simulink model "SVFB_notclean"  (R2024a)
settings: Solver=ode45  StartTime=0.0  StopTime=3  RelTol=1e-3
undefined symbols (not defined in the file): A, B, C, closed_loop_dynamics, closed_loop_observer, K0, L_luemb, S0_x0, Si_x0
settings Model: Creator=aless  LastModifiedBy=Stefano

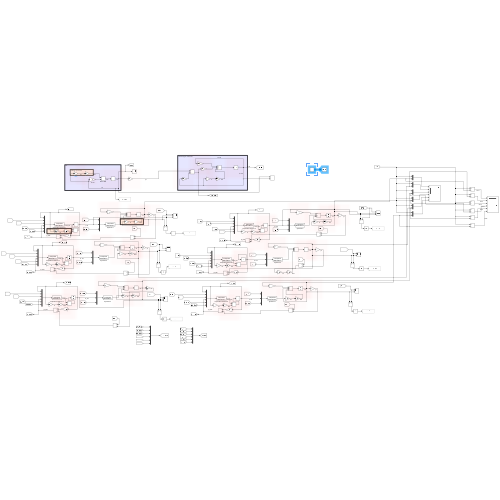
[thumbnail: Simulink's stored preview of the top-level diagram]
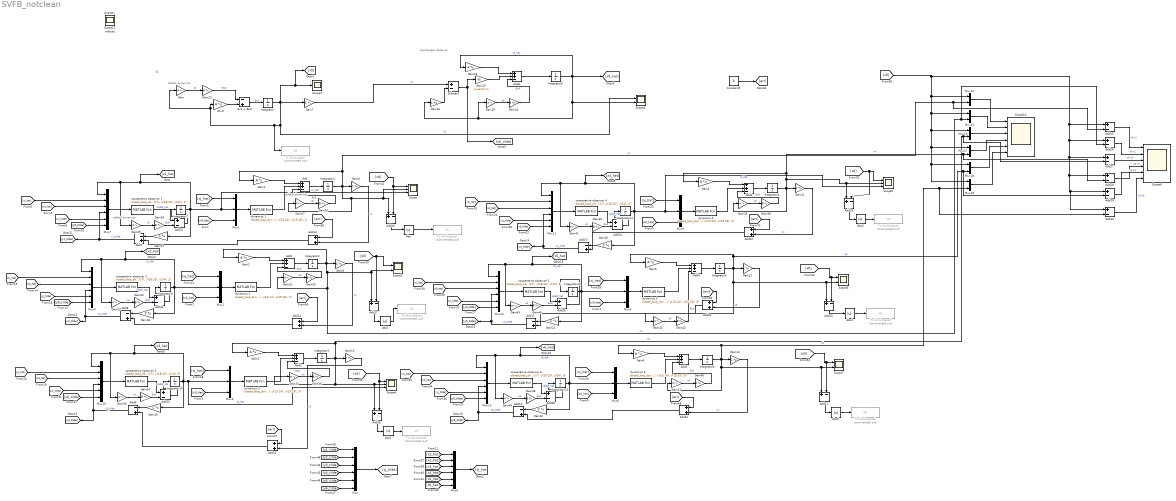
== system SVFB_notclean ==
  note: luemberger observer
  note: S0
  note: added dynamics
  note: added dynamics
  note: added dynamics
  A*x0 : Gain  Gain=A  Multiplication=Matrix(K*u)
  Abs{,1..5} (6 alike) : Abs  SaturateOnIntegerOverflow=off
  Add{,1..6} (7 alike) : Sum  Inputs=++-
  Add{7..12} (6 alike) : Sum  Inputs=-+
  Add{13..15,22..24} (6 alike) : Sum
  Add{16..21,25..36} (18 alike) : Sum  Inputs=+-
  Ax0 + Bu0 : Sum  Inputs=-+
  Constant5 : Constant  Value=0
  Gain{,25,27,29,31,33,35,37,39,41,43,45,47,49} (14 alike) : Gain  Gain=K0  Multiplication=Matrix(K*u)
  Gain{1..6,14} (7 alike) : Gain  Gain=A  Multiplication=Matrix(K*u)
  Gain{7..13,16..22} (14 alike) : Gain  Gain=C  Multiplication=Matrix(K*u)
  Gain15 : Gain  Gain=L_luemb  Multiplication=Matrix(K*u)
  Gain{23..24,26,28,30,32,34,36,38,40,42,44,46,48} (14 alike) : Gain  Gain=B  Multiplication=Matrix(K*u)
  Integrator : Integrator  InitialCondition=S0_x0
  Integrator{1..7,9..13} (12 alike) : Integrator  InitialCondition=Si_x0
  Integrator8 : Integrator  InitialCondition=S0_x0
  Mux{,7..13} (8 alike) : Mux  Inputs=6
  Mux{1..6} (6 alike) : Mux  Inputs=3
  Mux{14..19} (6 alike) : Mux  Inputs=2
  Scope : Scope  NumInputPorts=3
  Scope1 : Scope
  Scope10 : Scope  NumInputPorts=6
  Scope{2..3,6..7} (4 alike) : Scope  NumInputPorts=2
  Scope4 : Scope  NumInputPorts=3
  Scope5 : Scope  NumInputPorts=3
  Scope8 : Scope  NumInputPorts=6
  Subtract : Sum  Inputs=+-
  To Workspace1 : ToWorkspace  Commented=on  VariableName=x1  SaveFormat=Timeseries  SampleTime=-1
  To Workspace2 : ToWorkspace  Commented=on  VariableName=x2  SaveFormat=Timeseries  SampleTime=-1
  To Workspace3 : ToWorkspace  Commented=on  VariableName=x3  SaveFormat=Timeseries  SampleTime=-1
  To Workspace4 : ToWorkspace  Commented=on  VariableName=x4  SaveFormat=Timeseries  SampleTime=-1
  To Workspace5 : ToWorkspace  Commented=on  VariableName=x5  SaveFormat=Timeseries  SampleTime=-1
  To Workspace6 : ToWorkspace  Commented=on  VariableName=x6  SaveFormat=Timeseries  SampleTime=-1
  To Workspace7 : ToWorkspace  Commented=on  VariableName=x0  SampleTime=-1
  cooperative observer 1 : MATLABFcn  MATLABFcn=closed_loop_observer(u(1:2), u(3:14), u(15:16), u(17), u(18:23), u(24), 1)
  cooperative observer 2 : MATLABFcn  MATLABFcn=closed_loop_observer(u(1:2), u(3:14), u(15:16), u(17), u(18:23), u(24), 2)
  cooperative observer 3 : MATLABFcn  MATLABFcn=closed_loop_observer(u(1:2), u(3:14), u(15:16), u(17), u(18:23), u(24), 3)
  cooperative observer 4 : MATLABFcn  MATLABFcn=closed_loop_observer(u(1:2), u(3:14), u(15:16), u(17), u(18:23), u(24), 4)
  cooperative observer 5 : MATLABFcn  MATLABFcn=closed_loop_observer(u(1:2), u(3:14), u(15:16), u(17), u(18:23), u(24), 5)
  cooperative observer 6 : MATLABFcn  MATLABFcn=closed_loop_observer(u(1:2), u(3:14), u(15:16), u(17), u(18:23), u(24), 6)
  dynamics 1 : MATLABFcn  MATLABFcn=closed_loop_dynamics(u(1:12), u(13:14), u(15:16), 1)
  dynamics 2 : MATLABFcn  MATLABFcn=closed_loop_dynamics(u(1:12), u(13:14), u(15:16), 2)
  dynamics 3 : MATLABFcn  MATLABFcn=closed_loop_dynamics(u(1:12), u(13:14), u(15:16), 3)
  dynamics 4 : MATLABFcn  MATLABFcn=closed_loop_dynamics(u(1:12), u(13:14), u(15:16), 4)
  dynamics 5 : MATLABFcn  MATLABFcn=closed_loop_dynamics(u(1:12), u(13:14), u(15:16), 5)
  dynamics 6 : MATLABFcn  MATLABFcn=closed_loop_dynamics(u(1:12), u(13:14), u(15:16), 6)
  Scope11 : Scope
  position : Scope
  velocity : Scope
  wires:
  A*x0/1 -> Ax0 + Bu0/2
  Integrator8/1 -> Gain14/1, [x0_hat], Gain25/1, Gain16/1, Scope2/2  "x0_hat"
  Add6/1 -> Integrator8/1
  Gain7/1 -> Subtract/1  "y0"
  Gain15/1 -> Add6/2
  Subtract/1 -> [y0_tilde], Gain15/1
  Ax0 + Bu0/1 -> Integrator/1  "dx0"
  Integrator/1 -> [x0], Scope1/1, Gain7/1, Scope2/1, To Workspace7/1, Gain/1, A*x0/1  "x0"
  Gain14/1 -> Add6/1
  Gain16/1 -> Subtract/2
  Gain21/1 -> Add11/1
  Add12/1 -> [y6_tilde], Mux13/4  "y6_tilde"
  Add7/1 -> [y1_tilde], Mux7/4  "y1_tilde"
  [y5_tilde] -> Mux/5
  Gain19/1 -> Add9/1
  Gain22/1 -> Add12/1
  Mux10/1 -> cooperative observer 3/1
  [y0_tilde] -> Mux10/6
  Add2/1 -> Integrator3/1
  Integrator10/1 -> Gain19/1, [x3_hat], Gain35/1, Mux10/1, Scope4/3, Mux3/2  "x3_hat"
  [x0_hat] -> Mux3/3
  [x0_hat] -> Mux10/3
  Mux3/1 -> dynamics 3/1
  Integrator3/1 -> Add27/2, Mux16/2, Gain3/1, Gain37/1, Add18/1, Scope4/2, Gain10/1  "x3"
  dynamics 3/1 -> Add2/2
  [yj_tilde] -> Mux10/5
  Mux11/1 -> cooperative observer 4/1
  [xj_hat] -> Mux4/1
  Mux4/1 -> dynamics 4/1
  [y0_tilde] -> Mux11/6
  Gain3/1 -> Add2/1
  Integrator4/1 -> Gain11/1, Gain39/1, Add28/2, Mux17/2, Gain4/1, Add19/1, Scope5/2  "x4"
  Add3/1 -> Integrator4/1
  Integrator11/1 -> Gain20/1, [x4_hat], Gain41/1, Mux11/1, Scope5/3, Mux4/2  "x4_hat"
  dynamics 4/1 -> Add3/2
  Gain4/1 -> Add3/1
  [yj_tilde] -> Mux11/5
  Mux12/1 -> cooperative observer 5/1
  [xj_hat] -> Mux5/1
  Add4/1 -> Integrator5/1
  Integrator12/1 -> Gain21/1, [x5_hat], Gain45/1, Mux12/1, Mux5/2  "x5_hat"
  [x0_hat] -> Mux12/3
  dynamics 5/1 -> Add4/2
  Integrator5/1 -> Gain43/1, Scope6/2, Add20/1, Add29/2, Mux18/2, Gain5/1, Gain12/1  "x5"
  [xj_hat] -> Mux12/2
  [x0_hat] -> Mux5/3
  [yj_tilde] -> Mux12/5
  [x5_hat] -> Mux8/5
  [x3_hat] -> Mux8/3
  [x0_hat] -> Mux11/3
  [x2_hat] -> Mux8/2
  Gain18/1 -> Add8/1
  [yj_tilde] -> Mux9/5
  dynamics 2/1 -> Add1/2
  Gain2/1 -> Add1/1
  Integrator2/1 -> Gain31/1, Add26/2, Mux15/2, Scope3/2, Add17/1, Gain2/1, Gain9/1  "x2"
  Add10/1 -> Mux11/4, [y4_tilde]  "y4_tilde"
  Mux2/1 -> dynamics 2/1
  Gain5/1 -> Add4/1
  [x0_hat] -> Mux9/3
  [x0_hat] -> Mux2/3
  [xj_hat] -> Mux9/2
  Add11/1 -> Mux12/4, [y5_tilde]  "y5_tilde"
  [xj_hat] -> Mux2/1
  [y0_tilde] -> Mux9/6
  Integrator9/1 -> Gain18/1, [x2_hat], Gain33/1, Mux9/1, Mux2/2  "x2_hat"
  Add1/1 -> Integrator2/1
  Add5/1 -> Integrator6/1
  Mux13/1 -> cooperative observer 6/1
  [x0_hat] -> Mux4/3
  Integrator13/1 -> Gain22/1, [x6_hat], Gain49/1, Mux13/1, Mux6/2  "x6_hat"
  [x0_hat] -> Mux6/3
  [y0_tilde] -> Mux13/6
  Mux9/1 -> cooperative observer 2/1
  Mux6/1 -> dynamics 6/1
  [xj_hat] -> Mux6/1
  Integrator6/1 -> Gain47/1, Add21/1, Scope7/2, Add30/2, Mux19/2, Gain6/1, Gain13/1  "x6"
  Gain20/1 -> Add10/1
  [x6_hat] -> Mux8/6
  [y6_tilde] -> Mux/6
  Add8/1 -> [y2_tilde], Mux9/4  "y2_tilde"
  [yj_tilde] -> Mux13/5
  [y4_tilde] -> Mux/4
  Add9/1 -> [y3_tilde], Mux10/4  "y3_tilde"
  [y1_tilde] -> Mux/1
  Gain6/1 -> Add5/1
  Mux5/1 -> dynamics 5/1
  Mux7/1 -> cooperative observer 1/1
  [y3_tilde] -> Mux/3
  [y0_tilde] -> Mux12/6
  [xj_hat] -> Mux7/2
  [xj_hat] -> Mux3/1
  [x0_hat] -> Mux1/3
  [y0_tilde] -> Mux7/6
  Gain17/1 -> Add7/1
  [xj_hat] -> Mux1/1
  Mux8/1 -> [xj_hat]
  [x1_hat] -> Mux8/1
  [y2_tilde] -> Mux/2
  dynamics 6/1 -> Add5/2
  Integrator7/1 -> Gain17/1, [x1_hat], Gain29/1, Mux7/1, Scope/3, Mux1/2  "x1_hat"
  [xj_hat] -> Mux13/2
  [x0] -> Scope/1, Add16/2
  [xj_hat] -> Mux10/2
  [x0_hat] -> Mux7/3
  Integrator1/1 -> Gain27/1, Add16/1, Scope/2, Add25/2, Mux14/2, Gain1/1, Gain8/1  "x1"
  dynamics 1/1 -> Add/2
  [x4_hat] -> Mux8/4
  Add/1 -> Integrator1/1
  [x0_hat] -> Mux13/3
  Mux1/1 -> dynamics 1/1
  Gain1/1 -> Add/1
  [xj_hat] -> Mux11/2
  [yj_tilde] -> Mux7/5
  [x0] -> Scope3/1, Add17/2
  [x0] -> Add18/2, Scope4/1
  [x0] -> Add19/2, Scope5/1
  [x0] -> Scope6/1, Add20/2
  [x0] -> Add21/2, Scope7/1
  Mux/1 -> [yj_tilde]
  Mux14/1 -> Scope10/1
  Mux15/1 -> Scope10/2
  Mux16/1 -> Scope10/3
  Mux17/1 -> Scope10/4
  Mux18/1 -> Scope10/5
  Mux19/1 -> Scope10/6
  [x0] -> Add30/1, Add29/1, Add28/1, Add27/1, Add26/1, Add25/1, Mux19/1, Mux18/1, Mux17/1, Mux16/1, Mux15/1, Mux14/1
  Add16/1 -> Abs/1
  Abs/1 -> To Workspace1/1
  Add17/1 -> Abs1/1
  Abs1/1 -> To Workspace2/1
  Add18/1 -> Abs2/1
  Abs2/1 -> To Workspace3/1
  Add19/1 -> Abs3/1
  Abs3/1 -> To Workspace4/1
  Add20/1 -> Abs4/1
  Abs4/1 -> To Workspace5/1
  Add21/1 -> Abs5/1
  Abs5/1 -> To Workspace6/1
  Add13/1 -> Add7/2
  Gain8/1 -> Add13/2  "y1"
  Gain9/1 -> Add14/2  "y2"
  Add14/1 -> Add8/2
  Gain10/1 -> Add15/2  "y3"
  Add15/1 -> Add9/2
  Add22/1 -> Add10/2
  Gain11/1 -> Add22/2  "y4"
  Gain12/1 -> Add23/2  "y5"
  Add23/1 -> Add11/2
  Gain13/1 -> Add24/2  "y1"
  Add24/1 -> Add12/2
  Constant5/1 -> [err]
  [err] -> Add13/1
  [err] -> Add14/1
  [err] -> Add15/1
  [err] -> Add24/1
  [err] -> Add23/1
  [err] -> Add22/1
  Add26/1 -> Scope8/2  "x0-x2"
  Add25/1 -> Scope8/1  "x0-x1"
  Add29/1 -> Scope8/5  "x0-x5"
  Add30/1 -> Scope8/6  "x0-x6"
  Add27/1 -> Scope8/3  "x0-x3"
  Add28/1 -> Scope8/4  "x0-x4"
  Gain/1 -> Gain23/1  "u0"
  Gain23/1 -> Ax0 + Bu0/1  "Bu0"
  Gain24/1 -> Add6/3  "Bu0"
  Gain25/1 -> Gain24/1  "u0"
  Gain27/1 -> Gain26/1  "u0"
  Gain26/1 -> Add/3  "Bu0"
  Gain29/1 -> Gain28/1  "u0"
  cooperative observer 1/1 -> Add31/1  "x1dot_hat"
  Add31/1 -> Integrator7/1
  Gain28/1 -> Add31/2  "Bu0"
  Gain31/1 -> Gain30/1  "u0"
  Gain30/1 -> Add1/3  "Bu0"
  Gain32/1 -> Add32/2  "Bu0"
  Gain33/1 -> Gain32/1  "u0"
  cooperative observer 2/1 -> Add32/1  "x2dot_hat"
  Add32/1 -> Integrator9/1
  Gain34/1 -> Add33/2  "Bu0"
  Gain35/1 -> Gain34/1  "u0"
  cooperative observer 3/1 -> Add33/1  "x3dot_hat"
  Add33/1 -> Integrator10/1
  Gain37/1 -> Gain36/1  "u0"
  Gain36/1 -> Add2/3  "Bu0"
  Gain39/1 -> Gain38/1  "u0"
  Gain38/1 -> Add3/3  "Bu0"
  Gain40/1 -> Add34/2  "Bu0"
  Gain41/1 -> Gain40/1  "u0"
  cooperative observer 4/1 -> Add34/1  "x4dot_hat"
  Add34/1 -> Integrator11/1
  Gain43/1 -> Gain42/1  "u0"
  Gain42/1 -> Add4/3  "Bu0"
  Gain44/1 -> Add35/2  "Bu0"
  Gain45/1 -> Gain44/1  "u0"
  cooperative observer 5/1 -> Add35/1  "x5dot_hat"
  Add35/1 -> Integrator12/1
  Gain47/1 -> Gain46/1  "u0"
  Gain46/1 -> Add5/3  "Bu0"
  Gain48/1 -> Add36/2  "Bu0"
  Gain49/1 -> Gain48/1  "u0"
  cooperative observer 6/1 -> Add36/1  "x6dot_hat"
  Add36/1 -> Integrator13/1
